simulink model "Aplicacion"  (Simulink 9.1)
settings: Solver=ode45  StartTime=0.0  StopTime=10  RelTol=1e-3  AbsTol=1e-6
undefined symbols (not defined in the file or in its folder): sfunxy2
libraries: neural x1
settings Model: SuppressorTable=22 serialization::archive 11 0 6 0 0 0 1 0  Creator=matthew  LastModifiedBy=daniel  ExtModeTrigMode=oneshot  ExtModeArmWhenConnect=off  TunableVars=prueba  TunableVarsStorageClass=Auto
settings SolverCC: AutoScaleAbsTol=off
settings DataIOCC: SignalLoggingSaveFormat=ModelDataLogs  SaveOutput=off  SignalLoggingName=sigsOut
settings OptimizationCC: BooleanDataType=off  InitFltsAndDblsToZero=on
settings DebuggingCC: SaveWithParameterizedLinksMsg=none  SignalResolutionControl=TryResolveAllWithWarning  MultiTaskDSMMsg=warning  MultiTaskCondExecSysMsg=none
settings HardwareCC: TargetUnknown=on
settings RTWCC: TemplateMakefile=grt_vc.tmf
settings GRTTargetCC: TargetFcnLib=ansi_tfl_tmw.mat

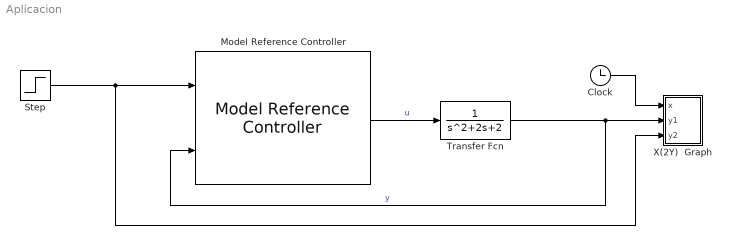
== system Aplicacion ==
  Clock : Clock
  Model Reference Controller : neural/Control Systems/Model Reference Controller  Nrc=2  Nic=2  Njc=2  IW_y=[-31.932093027544734554 -20.776392159179344787;-15.503407963641970824 -8.5944505816355292183;-1.9798404543843579617 20.220136489306408833;-2.1797825605546266026 -3.2841881188518331491]  IW_u=[14.956883661072257752 3.8896983118752839204;2.2058220589459600625 4.2659730499572035001;14.620364457568788552 14.820173646933977096;-9.4033189303473410092 8.7867015709859064287]  IW_r=[12.282614762626227645 13.833659857590200559;16.906978510992754394 15.72308775977682771;-0.85468072114202697787 -2.437652484521989571;0.1754720214355162955 -0.13545995920120590394]  B1_c=[-1.7406885184584026671;-19.248709423821647846;-6.6065936075787012882;-3.1217859320248395605]  B2_c=86.946382711951358147  LW_c=[100.01355776582298063 161.29107629728022744 87.085597291982779211 -87.600024717819238163]  retraining_c=2  max_i_int=10  min_i_int=1  max_r_int=10  min_r_int=1  Ts=0.05  S1=5  Ni=2  Nj=2  sim_file=ModeloPlanta  trainfun=trainlm  Use_validation=0  Use_Testing=0  Use_Inc_training=0  Use_previous_weights=1  max_i=4  min_i=0  max_r=2  min_r=0  sam_training=800  sam_training_c=800  epochs=300  epochs_c=20  minp=0.11732937101744811415  maxp=3.8920544955712816915  mint=0  maxt=3.8920544955712816915  Normalize=0  IW=[-0.00068315878223644218616 2.2983194652314774492e-05;-4.8840510221127967944e-05 -0.0001245082391853258503;0.14141180019962437675 -0.57090832612459485595;-0.00021595568732164237865 0.0016293115672855915891;-0.069595846475342199033 0.34643987842630363794]  LW1_2=[-0.29312765773512405865 0.17156559478486652082;0.21152458438154492226 -0.10901385675686174614;-0.89865501164796468547 1.3181002252571905053;0.23955622198751913565 -0.088627773486048763707;1.4212630256626264114 -1.7808562323093335422]  LW2_1=[-6.4581286690600583356 8.5409607712295763093 -0.13198233103366660557 2.1410315361998151218 -0.18960605208037734082]  B1=[-0.42502570815678153426;-1.5302054253162018504;0.040934612844617357386;-0.81643280624545633284;0.061038405543512634643]  B2=6.6425199390193894189  S1c=4  Limit_output=0  min_output=-Inf  max_output=Inf  Ref_file=ModeloPlantaReferencia
      settings: SourceProductName=Neural Network Toolbox  SourceProductBaseCode=NN
  Step : Step  Time=0  SampleTime=0
  Transfer Fcn : TransferFcn  Denominator=[1 2 2]
  X(2Y)  Graph : Subsystem  LoadFcn=sfunxy2([],[],[],'LoadBlock')  StartFcn=sfunxy2([],[],[],'Start')  StopFcn=sfunxy2([],[],[],'Stop')  mask(X(2Y) scope.){xmin=0, xmax=10, ymin=0, ymax=2, st=-1}
      mask prompts: xmin "x-min:"; xmax "x-max:"; ymin "y-min:"; ymax "y-max:"; st "Sample time:"
      mask help: X(2Y) scope using MATLAB graph window. First input is used as time base. Enter plotting ranges.
      settings: CopyFcn=sfunxy2([],[],[],'CopyBlock')  DeleteFcn=sfunxy2([],[],[],'DeleteBlock')  NameChangeFcn=sfunxy2([],[],[],'NameChange')
      mask Help: This block can be used to explore limit cycles. Look at the m-file sfunxy.m to see how it works.
      mask Display: plot([.05 .95 .95 .05 .05],[.45 .45 .95 .95 .45], 0.5+cos(0:0.1:2*pi)*0.3,0.7+sin(0:0.1:2*pi)*0.2)
  wires:
  Transfer Fcn/1 -> X(2Y)  Graph/2(y1), Model Reference Controller/2  "y"
  Model Reference Controller/1 -> Transfer Fcn/1  "u"
  Clock/1 -> X(2Y)  Graph/1(x)
  Step/1 -> X(2Y)  Graph/3(y2), Model Reference Controller/1

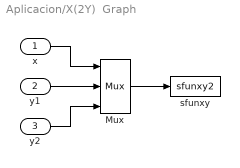
== system Aplicacion/X(2Y)  Graph ==
  x : Inport
  y1 : Inport  Port=2
  y2 : Inport  Port=3
  Mux : Mux  Inputs=3
  sfunxy : S-Function  FunctionName=sfunxy2  Parameters=[xmin xmax ymin ymax], st  SFunctionDeploymentMode=off  EnableBusSupport=off
  wires:
  y2/1 -> Mux/3
  y1/1 -> Mux/2
  x/1 -> Mux/1
  Mux/1 -> sfunxy/1
